simulink model "controller"  (R2018b)
settings: Solver=VariableStepAuto  StartTime=0.0  StopTime=10.0  RelTol=1e-3
settings Model: Creator=pthb3  LastModifiedBy=pthb3

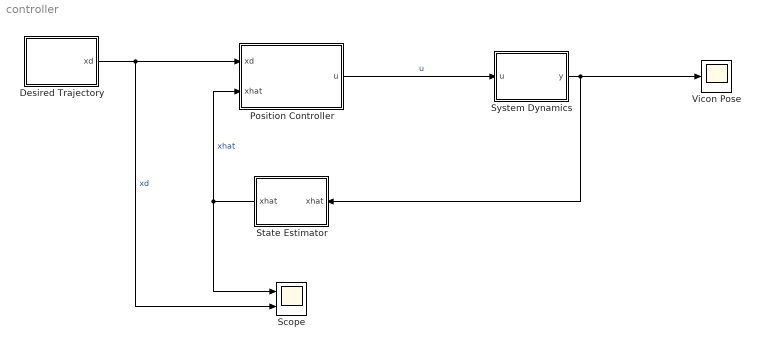
== system controller ==
  Desired Trajectory : MATLAB Function  TreatAsAtomicUnit=on
  Position Controller : MATLAB Function  TreatAsAtomicUnit=on
  Scope : Scope  NumInputPorts=2
  State Estimator : MATLAB Function  TreatAsAtomicUnit=on
  System Dynamics : MATLAB Function  TreatAsAtomicUnit=on
  Vicon Pose : Scope
  wires:
  Desired Trajectory/1(xd) -> Scope/2, Position Controller/1(xd)  "xd"
  Position Controller/1(u) -> System Dynamics/1(u)  "u"
  State Estimator/1(xhat) -> Scope/1, Position Controller/2(xhat)  "xhat"
  System Dynamics/1(y) -> Vicon Pose/1, State Estimator/1("xhat ")

== matlab function controller/Position Controller ==
  data: xd input; u output; xhat input
function u = controller(xd,xhat)

error = xd- xhat;
u = K * error;

== matlab function controller/Desired Trajectory ==
  data: xd output
function xd = trajectory()

xd = 1;

== matlab function controller/System Dynamics ==
  data: u input; y output
function y = plant(u)


y = A

y = u;

== matlab function controller/State Estimator ==
  data: xhat input; xhat output
function xhat = estimator(xhat)

xhat = y;
